simulink model "MATLAB_Func_u"  (R2020b)
settings: Solver=VariableStepAuto  StartTime=0.0  StopTime=10.0  RelTol=1e-3
settings Model: Creator=ShiningDanyang  LastModifiedBy=ShiningDanyang

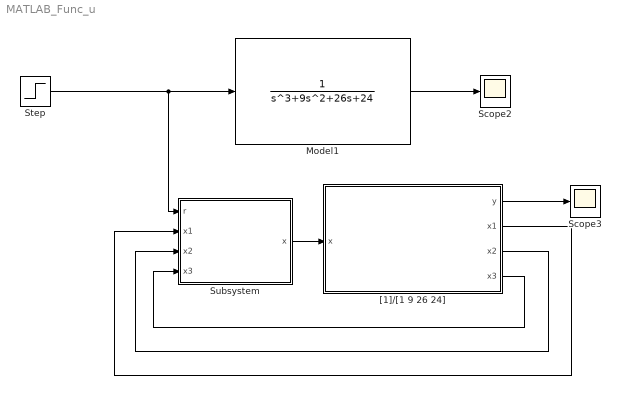
== system MATLAB_Func_u ==
  Model1 : TransferFcn  Denominator=[1 9 26 24]
  Scope2 : Scope
  Scope3 : Scope
  Step : Step  SampleTime=0
  Subsystem : Subsystem
  "[1]/[1 9 26 24]" : Subsystem
  wires:
  Step/1 -> Subsystem/1(r), Model1/1
  "[1]/[1 9 26 24]"/1(y) -> Scope3/1
  Model1/1 -> Scope2/1
  Subsystem/1(x) -> "[1]/[1 9 26 24]"/1(x)
  "[1]/[1 9 26 24]"/2(x1) -> Subsystem/2(x1)
  "[1]/[1 9 26 24]"/3(x2) -> Subsystem/3(x2)
  "[1]/[1 9 26 24]"/4(x3) -> Subsystem/4(x3)

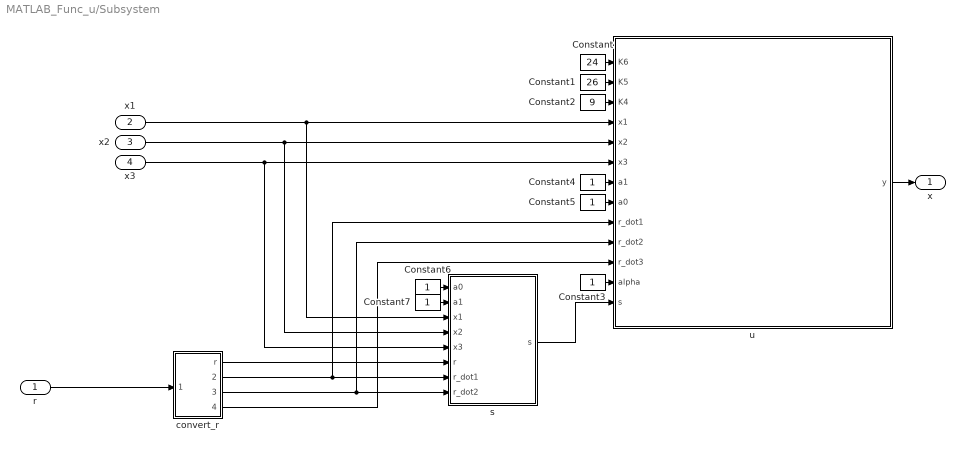
== system MATLAB_Func_u/Subsystem ==
  r : Inport
  x1 : Inport  Port=2
  x2 : Inport  Port=3
  x3 : Inport  Port=4
  Constant : Constant  Value=24
  Constant1 : Constant  Value=26
  Constant2 : Constant  Value=9
  Constant{3..7} (5 alike) : Constant
  convert_r : Subsystem
  s : MATLAB Function  TreatAsAtomicUnit=on
  u : MATLAB Function  TreatAsAtomicUnit=on
  x : Outport
  wires:
  convert_r/4(r_dot3) -> u/11(r_dot3)
  convert_r/3(r_dot2) -> u/10(r_dot2), s/8(r_dot2)
  Constant5/1 -> u/8(a0)
  Constant7/1 -> s/2(a1)
  convert_r/2(r_dot1) -> u/9(r_dot1), s/7(r_dot1)
  Constant1/1 -> u/2(K5)
  Constant2/1 -> u/3(K4)
  Constant6/1 -> s/1(a0)
  Constant/1 -> u/1(K6)
  Constant4/1 -> u/7(a1)
  Constant3/1 -> u/12(alpha)
  convert_r/1(r) -> s/6(r)
  r/1 -> convert_r/1(r_raw)
  s/1(s) -> u/13(s)
  x1/1 -> s/3(x1), u/4(x1)
  x2/1 -> s/4(x2), u/5(x2)
  x3/1 -> s/5(x3), u/6(x3)
  u/1(y) -> x/1

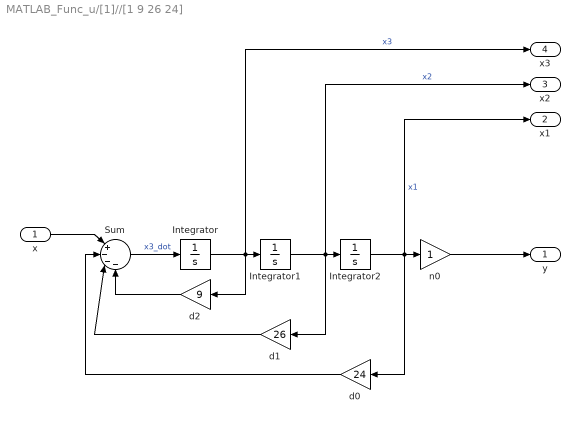
== system MATLAB_Func_u/[1]//[1 9 26 24] ==
  x : Inport
  Integrator : Integrator
  Integrator1 : Integrator
  Integrator2 : Integrator
  Sum : Sum  Inputs=|+---
  d0 : Gain  Gain=24
  d1 : Gain  Gain=26
  d2 : Gain  Gain=9
  n0 : Gain
  y : Outport
  x1 : Outport  Port=2
  x2 : Outport  Port=3
  x3 : Outport  Port=4
  wires:
  d0/1 -> Sum/2
  Sum/1 -> Integrator/1  "x3_dot"
  Integrator1/1 -> x2/1, d1/1, Integrator2/1  "x2"
  d2/1 -> Sum/4
  Integrator2/1 -> x1/1, d0/1, n0/1  "x1"
  Integrator/1 -> x3/1, d2/1, Integrator1/1  "x3"
  d1/1 -> Sum/3
  x/1 -> Sum/1
  n0/1 -> y/1

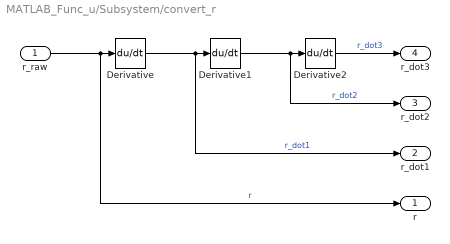
== system MATLAB_Func_u/Subsystem/convert_r ==
  r_raw : Inport
  Derivative : Derivative
  Derivative1 : Derivative
  Derivative2 : Derivative
  r : Outport
  r_dot1 : Outport  Port=2
  r_dot2 : Outport  Port=3
  r_dot3 : Outport  Port=4
  wires:
  Derivative1/1 -> r_dot2/1, Derivative2/1  "r_dot2"
  Derivative/1 -> r_dot1/1, Derivative1/1  "r_dot1"
  r_raw/1 -> r/1, Derivative/1  "r"
  Derivative2/1 -> r_dot3/1  "r_dot3"

== matlab function MATLAB_Func_u/Subsystem/s ==
  data: a0 input; s output; a1 input; x1 input; x2 input; x3 input; r input; r_dot1 input; r_dot2 input
function s = fcn(a0, a1, x1, x2, x3, r, r_dot1, r_dot2)
    s = x3 + a1*x2 + a0*x1 - (r_dot2 + a1*r_dot1 + a0*r);
end

== matlab function MATLAB_Func_u/Subsystem/u ==
  data: K6 input; y output; K5 input; K4 input; x1 input; x2 input; x3 input; a1 input; a0 input; r_dot1 input; r_dot2 input; r_dot3 input; alpha input; s input
function y = fcn(K6, K5, K4, x1, x2, x3, a1, a0, r_dot1, r_dot2, r_dot3, alpha, s)
    y = -(-K6*x1 -K5*x2 - K4*x3 + a1*(x3 - r_dot2) + a0*(x2 - r_dot1) - r_dot3 + alpha*sign(s));
end
